simulink library "INT_SyC_Main"  (R2016b)
settings: Solver=VariableStepAuto  StartTime=0.0  StopTime=10.0  RelTol=1e-3
settings Model: Creator=liutao  LastModifiedBy=liutao

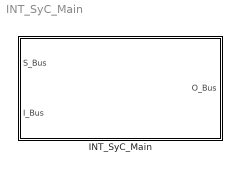
== system INT_SyC_Main ==
  INT_SyC_Main : Subsystem

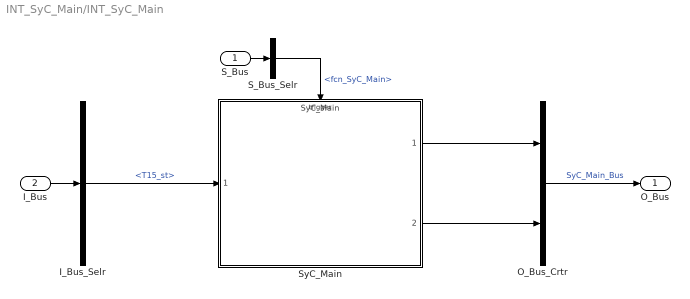
== system INT_SyC_Main/INT_SyC_Main ==
  S_Bus : Inport
  I_Bus : Inport  Port=2
  I_Bus_Selr : BusSelector  OutputSignals=T15_st
  O_Bus_Crtr : BusCreator  Inputs=2
  S_Bus_Selr : BusSelector  OutputSignals=fcn_SyC_Main
  SyC_Main : ModelReference  ModelNameDialog=SyC_Main  SimulationMode=Normal  ModelReferenceVersion=1.10  TriggerPortName=function  TriggerPortTriggerType=function-call  TriggerPortStatesWhenEnabling=held
  O_Bus : Outport
  wires:
  S_Bus_Selr/1 -> SyC_Main/Trigger  "<fcn_SyC_Main>"
  S_Bus/1 -> S_Bus_Selr/1
  I_Bus/1 -> I_Bus_Selr/1
  I_Bus_Selr/1 -> SyC_Main/1  "<T15_st>"
  O_Bus_Crtr/1 -> O_Bus/1  "SyC_Main_Bus"
  SyC_Main/1 -> O_Bus_Crtr/1
  SyC_Main/2 -> O_Bus_Crtr/2
